simulink library "findPosition_ul"  (R2018b)
settings: Solver=VariableStepAuto  StartTime=0.0  StopTime=10.0  RelTol=1e-3
settings Model: Creator=mcobb  LastModifiedBy=MAE-NCSUCORE
settings DebuggingCC: LibraryContextMissingDiagnostic=none
settings SFSimCC: SimUseLocalCustomCode=off
settings RTWCC: RTWUseLocalCustomCode=off

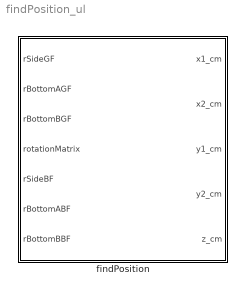
== system findPosition_ul ==
  findPosition : Subsystem

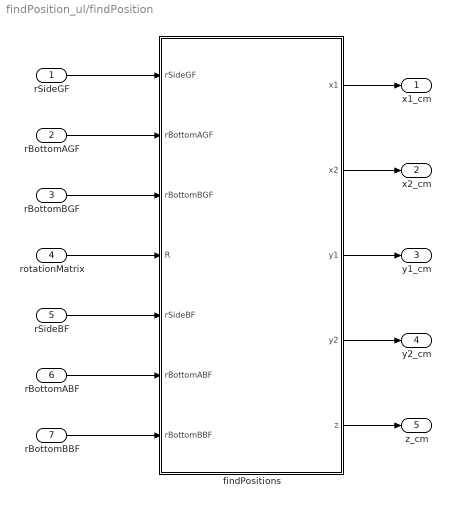
== system findPosition_ul/findPosition ==
  rSideGF : Inport
  rBottomAGF : Inport  Port=2
  rBottomBGF : Inport  Port=3
  rotationMatrix : Inport  Port=4
  rSideBF : Inport  Port=5
  rBottomABF : Inport  Port=6
  rBottomBBF : Inport  Port=7
  findPositions : MATLAB Function  TreatAsAtomicUnit=on
  x1_cm : Outport
  x2_cm : Outport  Port=2
  y1_cm : Outport  Port=3
  y2_cm : Outport  Port=4
  z_cm : Outport  Port=5
  wires:
  rSideGF/1 -> findPositions/1(rSideGF)
  rBottomAGF/1 -> findPositions/2(rBottomAGF)
  rBottomBGF/1 -> findPositions/3(rBottomBGF)
  rotationMatrix/1 -> findPositions/4(R)
  findPositions/1(x1) -> x1_cm/1
  findPositions/2(x2) -> x2_cm/1
  findPositions/3(y1) -> y1_cm/1
  findPositions/4(y2) -> y2_cm/1
  findPositions/5(z) -> z_cm/1
  rSideBF/1 -> findPositions/5(rSideBF)
  rBottomABF/1 -> findPositions/6(rBottomABF)
  rBottomBBF/1 -> findPositions/7(rBottomBBF)

== matlab function findPosition_ul/findPosition/findPositions ==
  data: x1 output; x2 output; rSideGF input; y1 output; y2 output; rBottomAGF input; rBottomBGF input; R input; rSideBF input; rBottomABF input; rBottomBBF input; z output
function [x1,x2,y1,y2,z] = ...
    fcn(rSideGF,rBottomAGF,rBottomBGF,R,rSideBF,rBottomABF,rBottomBBF)
%#codegen
[x1,x2,y1,y2,z] = ...
    findPosition(rSideGF,rBottomAGF,rBottomBGF,R,rSideBF,rBottomABF,rBottomBBF);
